simulink model "motor_eccentricity_fault"  (R2025a)
settings: Solver=FixedStepAuto  StartTime=0  StopTime=5  FixedStep=1e-4  RelTol=1e-3
undefined symbols (not defined in the file): f_supply, fault_severity, Torque_in, V_in
libraries: spsAsynchronousMachineSIUnitsLib x1, spsThreePhaseSourceLib x1, spspowerguiLib x1
settings Model: Creator=User  LastModifiedBy=User
settings DataIOCC: SaveOutput=off  DSMLogging=off  ReturnWorkspaceOutputs=off

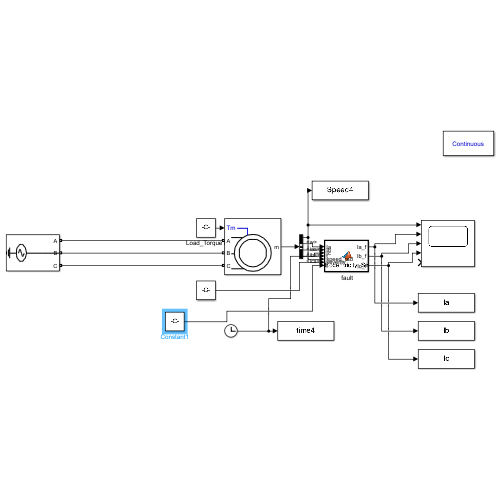
[thumbnail: Simulink's stored preview of the top-level diagram]
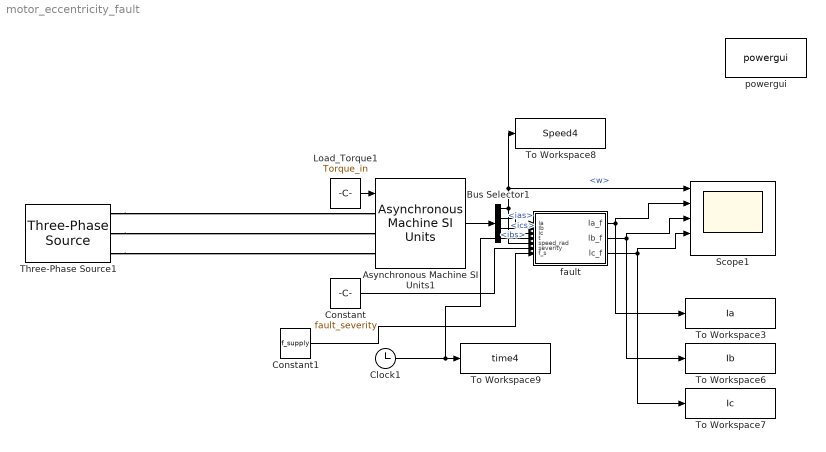
== system motor_eccentricity_fault ==
  " fault" : MATLAB Function  TreatAsAtomicUnit=on
  Asynchronous Machine SI Units1 : spsAsynchronousMachineSIUnitsLib/Asynchronous Machine SI Units  RotorType=Squirrel-cage  PresetModel=No  MechanicalLoad=Torque Tm  ShowDetailedParameters=on  ReferenceFrame=Stationary  Units=SI  MeasurementBus=on  NominalParameters=[7500 400 50]  VoltageRatio=1  Stator=[1.405 0.005839]  Rotor=[2 0.006839]  Cage1=[0.4155 0.002066]  Cage2=[0.4168 0.0003495]  Lm=0.1722  Mechanical=[0.0131 0.001 2]  PolePairs=2  InitialConditions=[0 0 0 0 0 0 0 0]  SimulateSaturation=off  Saturation=[14.03593122, 27.81365428, 53.79336849, 72.68890987, 97.98006896, 148.6815601, 215.7428561, 302.9841135, 428.7778367 ; 230, 322, 414, 460, 506, 552, 598, 644, 690]  LoadFlowParameters=1492000  TsPowergui=0  TsBlock=-1  IterativeModel=Trapezoidal non iterative  IterativeDiscreteModel=Trapezoidal non iterative  Pmec=1.492e+006
  Bus Selector1 : BusSelector  OutputSignals=w,ias,ibs,ics
  Clock1 : Clock
  Constant : Constant  Value=fault_severity
  Constant1 : Constant  Value=f_supply
  Load_Torque1 : Constant  Value=Torque_in
  Scope1 : Scope  NumInputPorts=5
      settings: ActiveDisplayYMinimum=-0.049617664684487431  ActiveDisplayYMaximum=0.049617664684487604
  Three-Phase Source1 : spsThreePhaseSourceLib/Three-Phase Source  InternalConnection=Yg  VoltagePhases=on  Voltage=400  PhaseAngle=0  Voltage_phases=[V_in V_in V_in]/sqrt(3)  PhaseAngles_phases=[0 -120 +120]  Frequency=f_supply  NonIdealSource=off  SpecifyImpedance=off  Resistance=0.8929  Inductance=16.58e-3  ShortCircuitLevel=100e6  BaseVoltage=25e3  XRratio=7  BusType=swing  Pref=10e3  Qref=0  Prefabc=[10e3, 10e3, 10e3]  Qrefabc=[0, 0, 0]  Qmin=-inf  Qmax=inf
  To Workspace3 : ToWorkspace  VariableName=Ia  SampleTime=-1
  To Workspace6 : ToWorkspace  VariableName=Ib  SampleTime=-1
  To Workspace7 : ToWorkspace  VariableName=Ic  SampleTime=-1
  To Workspace8 : ToWorkspace  VariableName=Speed4  SampleTime=-1
  To Workspace9 : ToWorkspace  VariableName=time4  SampleTime=-1
  powergui : spspowerguiLib/powergui  Priority=1  SimulationMode=Continuous  SampleTime=50e-6  frequency=60  Iterations=50  frequencyindice=50  Pbase=100e6  ErrMax=1e-4  UnitsV=kV  UnitsW=MW  buscounter=0  FunctionMessages=off  echomessages=off  EnableUseOfTLC=off  CurrentSourceSwitches=off  DisableSnubberDevices=off  DisableRonSwitches=off  DisableVfSwitches=off  DisplayEquations=off  AutomaticDiscreteSolvers=off  SolverType=Tustin/Backward Euler (TBE)  Interpol=off  ExternalGateDelay=off  methode=off  Ts=100  x0status=blocks  SPID=on  SwTol=0  HookPort=off  NonlinearTolerance=1e-4  nMaxIteration=100  ContinueOnMaxIteration=off  RestoreLinks=warning  ResistiveCurrentMeasurement=off  Frange=[0:2:500]  Ylog=off  Xlog=on  ShowGrid=off  save=off  variable=ZData  structure=0  ZoomFFT=off  StartTime=0.0  cycles=1  DisplayStyle=1  fundamental=60  FreqAxis=off  MaxFrequency=1000  frequencyindicesteady=1  RmsSteady=1  display=off
  wires:
  Clock1/1 -> " fault"/4(t), To Workspace9/1
  Asynchronous Machine SI Units1/1 -> Bus Selector1/1
  Bus Selector1/1 -> To Workspace8/1, Scope1/1, " fault"/5(speed_rad)  "<w>"
  Load_Torque1/1 -> Asynchronous Machine SI Units1/1
  " fault"/1(Ia_f) -> Scope1/2, To Workspace3/1
  " fault"/2(Ib_f) -> Scope1/3, To Workspace6/1
  " fault"/3(Ic_f) -> Scope1/4, To Workspace7/1
  Bus Selector1/2 -> " fault"/1(Ia)  "<ias>"
  Bus Selector1/3 -> " fault"/2(Ib)  "<ibs>"
  Bus Selector1/4 -> " fault"/3(Ic)  "<ics>"
  Constant/1 -> " fault"/6(severity)
  Constant1/1 -> " fault"/7(f_s)
  connections:
  Three-Phase Source1/RConn2 -- Asynchronous Machine SI Units1/LConn2
  Three-Phase Source1/RConn1 -- Asynchronous Machine SI Units1/LConn1
  Three-Phase Source1/RConn3 -- Asynchronous Machine SI Units1/LConn3

== matlab function motor_eccentricity_fault/ fault ==
  data: Ia input; Ia_f output; Ib input; Ic input; t input; Ib_f output; Ic_f output; speed_rad input; severity input; f_s input
function [Ia_f, Ib_f, Ic_f] = MixedEccentricity_Simulink(...
    Ia, Ib, Ic, t, speed_rad, severity, f_s)
    %#codegen
    % MIXED ECCENTRICITY - FIXED for Simulink
    % Input sizes must be explicitly defined or inherited
    %
    % Inputs:
    %   Ia, Ib, Ic: Stator currents (scalar at each time step)
    %   speed_rpm: Rotor speed in RPM (scalar at each time step)
    %   t: Time (scalar)
    %   severity: Fault severity 0-1 (scalar parameter)
    %
    % Outputs:
    %   Ia_f, Ib_f, Ic_f: Faulty stator currents (same size as inputs)
    % Default motor parameters for your 7.5kVA motor
  
    speed_rpm = speed_rad * 9.549;
    % Ensure speed_rpm is scalar (handle both scalar and vector inputs)
    % If speed_rpm is a vector, use the first element
    if ~isscalar(speed_rpm)
        speed_rpm_val = speed_rpm(1);
    else
        speed_rpm_val = speed_rpm;
    end
    
    % Calculate rotor frequency (Hz)
    f_r = abs(speed_rpm_val) / 60.0;
    
    % Initialize outputs (pass through if no fault)
    Ia_f = Ia;
    Ib_f = Ib;
    Ic_f = Ic;
    
    % Only apply fault if severity > 0
    if severity > 0
        % Ensure f_lower is positive (avoid negative frequency)
        f_lower = max(0.1, f_s - f_r);
        f_upper = f_s + f_r;
        
        % Fault amplitude (adjust 1.5 based on your motor size)
        fault_amp = severity * 2.9;
        
        % Mixed eccentricity = 40% static + 60% dynamic
        static_component = fault_amp * 0.4 * sin(2.0 * pi * f_s * t);
        dynamic_component = fault_amp * 0.6 * (...
            sin(2.0 * pi * f_lower * t) + ...
            sin(2.0 * pi * f_upper * t));
        
        combined_fault = static_component + dynamic_component;
        
        % Apply to all phases
        Ia_f = Ia + combined_fault;
        Ib_f = Ib + combined_fault;
        Ic_f = Ic + combined_fault;
    end
end
